simulink model "Battery_Connected_3_Phase_GridTied_Inverter_r2019a"  (R2019a)
settings: Solver=ode3  StartTime=0.0  StopTime=4  FixedStep=dtsim  RelTol=1e-3
values from neighbouring files (symbols this model uses):
  a1_lpf = 1.3601/wc_lpf    (= 4.32933276199e-05)    [Battery_Connected_3_Phase_GridTied_Inverter_Parameters.m]    (also in NonDispDGParameters.m)
  a2_lpf = 0.6165/wc_lpf2    (= 6.24645097155e-10)    [Battery_Connected_3_Phase_GridTied_Inverter_Parameters.m]    (also in NonDispDGParameters.m)
  bf = 2 * eta * wc    [Battery_Connected_3_Phase_GridTied_Inverter_Parameters.m]    (also in NonDispDGParameters.m)
  C_HV = 100e-6    (= 0.0001)    [Battery_Connected_3_Phase_GridTied_Inverter_Parameters.m]    (also in NonDispDGParameters.m; power_converters_DAB_1ph_Parameters.m)
  C_LV = 2000e-6    (= 0.002)    [Battery_Connected_3_Phase_GridTied_Inverter_Parameters.m]    (also in NonDispDGParameters.m; power_converters_DAB_1ph_Parameters.m)
  Cdc = 2 * E_Cdc / Vdc / Vdc    (= 0.00125)    [Battery_Connected_3_Phase_GridTied_Inverter_Parameters.m]    (also in NonDispDGParameters.m)
  Cf = x*Cb    (= 7.95774715459e-06)    [Battery_Connected_3_Phase_GridTied_Inverter_Parameters.m]    (also in NonDispDGParameters.m = 8.72536076817e-06)
  cf = wc * wc    (= 15791.3670417)    [Battery_Connected_3_Phase_GridTied_Inverter_Parameters.m]    (also in NonDispDGParameters.m)
  Cs_FET = inf    [Battery_Connected_3_Phase_GridTied_Inverter_Parameters.m]    (also in NonDispDGParameters.m; power_converters_DAB_1ph_Parameters.m)
  dP1 = 0.3    [Battery_Connected_3_Phase_GridTied_Inverter_Parameters.m]    (also in NonDispDGParameters.m)
  dP2 = 0.5    [Battery_Connected_3_Phase_GridTied_Inverter_Parameters.m]    (also in NonDispDGParameters.m)
  dP3 = 0.8    [Battery_Connected_3_Phase_GridTied_Inverter_Parameters.m]    (also in NonDispDGParameters.m = 0.2)
  dP4 = -0.6    [Battery_Connected_3_Phase_GridTied_Inverter_Parameters.m]    (also in NonDispDGParameters.m)
  dtsim = 5.0e-6    (= 5e-06)    [Battery_Connected_3_Phase_GridTied_Inverter_Parameters.m]    (also in NonDispDGParameters.m)
  f0 = 50    [Battery_Connected_3_Phase_GridTied_Inverter_Parameters.m]    (also in NonDispDGParameters.m)
  Fsw = 10e3    (= 10000)    [Battery_Connected_3_Phase_GridTied_Inverter_Parameters.m]    (also in NonDispDGParameters.m; power_converters_DAB_1ph_Parameters.m = 5000)
  Ia_limit = 1    [Battery_Connected_3_Phase_GridTied_Inverter_Parameters.m]    (also in NonDispDGParameters.m)
  Ib_peak = Ib*sqrt(2)    [Battery_Connected_3_Phase_GridTied_Inverter_Parameters.m]    (also in NonDispDGParameters.m)
  Ir_limit = 1    [Battery_Connected_3_Phase_GridTied_Inverter_Parameters.m]    (also in NonDispDGParameters.m)
  Ki = Kp/Ti    [Battery_Connected_3_Phase_GridTied_Inverter_Parameters.m]    (also in NonDispDGParameters.m)
  Kii = (BW_conv/w0) * Rseries_pu * w0    [Battery_Connected_3_Phase_GridTied_Inverter_Parameters.m]    (also in NonDispDGParameters.m)
  Kip = BW_P    [Battery_Connected_3_Phase_GridTied_Inverter_Parameters.m]    (also in NonDispDGParameters.m)
  Kiq = BW_Q    [Battery_Connected_3_Phase_GridTied_Inverter_Parameters.m]    (also in NonDispDGParameters.m)
  Kp = 2/A0 * KP    [Battery_Connected_3_Phase_GridTied_Inverter_Parameters.m]    (also in NonDispDGParameters.m)
  Kpi = (BW_conv/w0) * Lseries_pu    [Battery_Connected_3_Phase_GridTied_Inverter_Parameters.m]    (also in NonDispDGParameters.m)
  Kpp = BW_P * Tconv    [Battery_Connected_3_Phase_GridTied_Inverter_Parameters.m]    (also in NonDispDGParameters.m)
  Kpq = BW_Q * Tconv    [Battery_Connected_3_Phase_GridTied_Inverter_Parameters.m]    (also in NonDispDGParameters.m)
  L_Inductor = 1000e-6    (= 0.001)    [Battery_Connected_3_Phase_GridTied_Inverter_Parameters.m]    (also in NonDispDGParameters.m; power_converters_DAB_1ph_Parameters.m = 8e-06)
  Lgrid = Xgrid/w0    (= 0.00795774715459)    [Battery_Connected_3_Phase_GridTied_Inverter_Parameters.m]    (also in NonDispDGParameters.m)
  Li = Vdc/(16*fsw*delta_Ilmax)    [Battery_Connected_3_Phase_GridTied_Inverter_Parameters.m]    (also in NonDispDGParameters.m)
  Li_pu = Li/Lb    [Battery_Connected_3_Phase_GridTied_Inverter_Parameters.m]    (also in NonDispDGParameters.m)
  Lm_Tr = 100e-3    (= 0.1)    [Battery_Connected_3_Phase_GridTied_Inverter_Parameters.m]    (also in NonDispDGParameters.m; power_converters_DAB_1ph_Parameters.m = 0.00072)
  Lprim_Tr = 1e-7    (= 1e-07)    [Battery_Connected_3_Phase_GridTied_Inverter_Parameters.m]    (also in NonDispDGParameters.m; power_converters_DAB_1ph_Parameters.m = 0)
  Lsec_Tr = 1e-7    (= 1e-07)    [Battery_Connected_3_Phase_GridTied_Inverter_Parameters.m]    (also in NonDispDGParameters.m; power_converters_DAB_1ph_Parameters.m = 1.7e-05)
  ma = E_ltl*sqrt(2)/Vdc    [Battery_Connected_3_Phase_GridTied_Inverter_Parameters.m]    (also in NonDispDGParameters.m)
  Ntran = Vmv/Vlv    (= 1.9)    [Battery_Connected_3_Phase_GridTied_Inverter_Parameters.m]    (also in NonDispDGParameters.m = 1.98952879581)
  phia = 0    [Battery_Connected_3_Phase_GridTied_Inverter_Parameters.m]    (also in NonDispDGParameters.m)
  Pinit = 0    [Battery_Connected_3_Phase_GridTied_Inverter_Parameters.m]    (also in NonDispDGParameters.m)
  Pnom = 1000    [Battery_Connected_3_Phase_GridTied_Inverter_Parameters.m]    (also in NonDispDGParameters.m; power_converters_DAB_1ph_Parameters.m = 10000)
  R_DCsrc1 = 1e-7    (= 1e-07)    [Battery_Connected_3_Phase_GridTied_Inverter_Parameters.m]    (also in NonDispDGParameters.m; power_converters_DAB_1ph_Parameters.m)
  R_Inductor = 16e-3    (= 0.016)    [Battery_Connected_3_Phase_GridTied_Inverter_Parameters.m]    (also in NonDispDGParameters.m; power_converters_DAB_1ph_Parameters.m)
  RC_HV = 1e-3    (= 0.001)    [Battery_Connected_3_Phase_GridTied_Inverter_Parameters.m]    (also in NonDispDGParameters.m; power_converters_DAB_1ph_Parameters.m)
  RC_LV = 1e-3    (= 0.001)    [Battery_Connected_3_Phase_GridTied_Inverter_Parameters.m]    (also in NonDispDGParameters.m; power_converters_DAB_1ph_Parameters.m)
  Rd = 1/(3*wres*Cf)    [Battery_Connected_3_Phase_GridTied_Inverter_Parameters.m]    (also in NonDispDGParameters.m)
  Rgrid = 0.7    [Battery_Connected_3_Phase_GridTied_Inverter_Parameters.m]    (also in NonDispDGParameters.m)
  Ri = Ri_pu*Zb    [Battery_Connected_3_Phase_GridTied_Inverter_Parameters.m]    (also in NonDispDGParameters.m)
  Rm_Tr = 1e6    (= 1000000)    [Battery_Connected_3_Phase_GridTied_Inverter_Parameters.m]    (also in NonDispDGParameters.m; power_converters_DAB_1ph_Parameters.m = 10000)
  Ron_Diode = 10e-3    (= 0.01)    [Battery_Connected_3_Phase_GridTied_Inverter_Parameters.m]    (also in NonDispDGParameters.m; power_converters_DAB_1ph_Parameters.m)
  Ron_FET = 20e-3    (= 0.02)    [Battery_Connected_3_Phase_GridTied_Inverter_Parameters.m]    (also in NonDispDGParameters.m; power_converters_DAB_1ph_Parameters.m = 0.016)
  Rprim_Tr = 10e-3    (= 0.01)    [Battery_Connected_3_Phase_GridTied_Inverter_Parameters.m]    (also in NonDispDGParameters.m; power_converters_DAB_1ph_Parameters.m = 1e-06)
  Rs_FET = 1e6    (= 1000000)    [Battery_Connected_3_Phase_GridTied_Inverter_Parameters.m]    (also in NonDispDGParameters.m; power_converters_DAB_1ph_Parameters.m)
  Rsec_Tr = 10e-3    (= 0.01)    [Battery_Connected_3_Phase_GridTied_Inverter_Parameters.m]    (also in NonDispDGParameters.m; power_converters_DAB_1ph_Parameters.m = 0.043)
  Rtran_pu = 0.003    [Battery_Connected_3_Phase_GridTied_Inverter_Parameters.m]    (also in NonDispDGParameters.m)
  Sb = Pinv    (= 1000)    [Battery_Connected_3_Phase_GridTied_Inverter_Parameters.m]    (also in NonDispDGParameters.m)
  Stran = 1000    [Battery_Connected_3_Phase_GridTied_Inverter_Parameters.m]    (also in NonDispDGParameters.m)
  tinit = 0.25    [Battery_Connected_3_Phase_GridTied_Inverter_Parameters.m]    (also in NonDispDGParameters.m)
  tP1 = 0.5    [Battery_Connected_3_Phase_GridTied_Inverter_Parameters.m]    (also in NonDispDGParameters.m)
  tP2 = 1.5    [Battery_Connected_3_Phase_GridTied_Inverter_Parameters.m]    (also in NonDispDGParameters.m)
  tP3 = 2.5    [Battery_Connected_3_Phase_GridTied_Inverter_Parameters.m]    (also in NonDispDGParameters.m)
  tP4 = 3.5    [Battery_Connected_3_Phase_GridTied_Inverter_Parameters.m]    (also in NonDispDGParameters.m)
  Ts = 1e-7    (= 1e-07)    [Battery_Connected_3_Phase_GridTied_Inverter_Parameters.m]    (also in NonDispDGParameters.m; power_converters_DAB_1ph_Parameters.m)
  Turn_ratio = 15    [Battery_Connected_3_Phase_GridTied_Inverter_Parameters.m]    (also in NonDispDGParameters.m; power_converters_DAB_1ph_Parameters.m)
  Vb_peak = Vb*sqrt(2/3)    [Battery_Connected_3_Phase_GridTied_Inverter_Parameters.m]    (also in NonDispDGParameters.m)
  Vbat = 25    [Battery_Connected_3_Phase_GridTied_Inverter_Parameters.m]    (also in NonDispDGParameters.m = 24; power_converters_DAB_1ph_Parameters.m = 24)
  Vc_prime = 0.25    [Battery_Connected_3_Phase_GridTied_Inverter_Parameters.m]    (also in NonDispDGParameters.m)
  Vdc = 400    [Battery_Connected_3_Phase_GridTied_Inverter_Parameters.m]    (also in NonDispDGParameters.m)
  Vf_Diode = 4.2    [Battery_Connected_3_Phase_GridTied_Inverter_Parameters.m]    (also in NonDispDGParameters.m; power_converters_DAB_1ph_Parameters.m)
  Vlv = 200    [Battery_Connected_3_Phase_GridTied_Inverter_Parameters.m]    (also in NonDispDGParameters.m = 191)
  Vmv = 380    [Battery_Connected_3_Phase_GridTied_Inverter_Parameters.m]    (also in NonDispDGParameters.m)
  w0 = 2*pi*f0    (= 314.159265359)    [Battery_Connected_3_Phase_GridTied_Inverter_Parameters.m]    (also in NonDispDGParameters.m)
  Xtran_pu = 0.6    [Battery_Connected_3_Phase_GridTied_Inverter_Parameters.m]    (also in NonDispDGParameters.m)
undefined symbols (not defined in the file or in its folder): D11, Delta, Ion, Lg, Lithium
libraries: powerlib x48, simulink x8, powerlib_meascontrol x4, simulink_extras x2, electricdrivelib x1
(part 2 of 2)

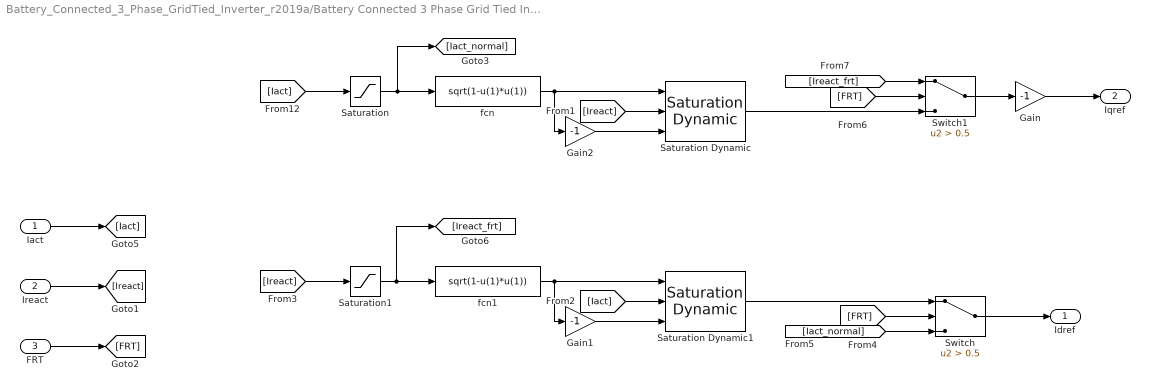
== system Battery_Connected_3_Phase_GridTied_Inverter_r2019a/Battery Connected 3 Phase Grid Tied Inverter/dq_limiter ==
  Iact : Inport
  Ireact : Inport  Port=2
  FRT : Inport  Port=3
  Gain : Gain  Gain=-1
  Gain1 : Gain  Gain=-1
  Gain2 : Gain  Gain=-1
  Saturation : Saturate  UpperLimit=1  LowerLimit=-1
  Saturation Dynamic : simulink/Discontinuities/Saturation Dynamic  OutMin=[]  OutMax=[]  OutDataTypeStr=Inherit: Same as second input  OutDataType=fixdt(1, 16)  OutScaling=2^-10  DoSatur=off
  Saturation Dynamic1 : simulink/Discontinuities/Saturation Dynamic  OutMin=[]  OutMax=[]  OutDataTypeStr=Inherit: Same as second input  OutDataType=fixdt(1, 16)  OutScaling=2^-10  DoSatur=off
  Saturation1 : Saturate  UpperLimit=1  LowerLimit=-1
  Switch : Switch  Criteria=u2 > Threshold  Threshold=0.5
  Switch1 : Switch  Criteria=u2 > Threshold  Threshold=0.5
  fcn : Fcn  Expr=sqrt(1-u(1)*u(1))
  fcn1 : Fcn  Expr=sqrt(1-u(1)*u(1))
  Idref : Outport  VectorParamsAs1DForOutWhenUnconnected=off
  Iqref : Outport  Port=2  VectorParamsAs1DForOutWhenUnconnected=off
  wires:
  fcn/1 -> Gain2/1, Saturation Dynamic/1
  Gain2/1 -> Saturation Dynamic/3
  Saturation/1 -> [Iact_normal], fcn/1
  Iact/1 -> [Iact]
  Ireact/1 -> [Ireact]
  [Iact] -> Saturation/1
  [Ireact] -> Saturation Dynamic/2
  [Iact] -> Saturation Dynamic1/2
  Gain1/1 -> Saturation Dynamic1/3
  fcn1/1 -> Gain1/1, Saturation Dynamic1/1
  [Ireact] -> Saturation1/1
  FRT/1 -> [FRT]
  [FRT] -> Switch/2
  Saturation Dynamic/1 -> Switch1/3
  Saturation1/1 -> [Ireact_frt], fcn1/1
  [Iact_normal] -> Switch/3
  Saturation Dynamic1/1 -> Switch/1
  Switch/1 -> Idref/1
  [FRT] -> Switch1/2
  [Ireact_frt] -> Switch1/1
  Switch1/1 -> Gain/1
  Gain/1 -> Iqref/1

== system Battery_Connected_3_Phase_GridTied_Inverter_r2019a/Battery Connected 3 Phase Grid Tied Inverter/dq_to_abc ==
  dq : Inport
  theta : Inport  Port=2
  Vdc : Inport  Port=3
  Divide : Product  Inputs=*/
  Mux2 : Mux  Inputs=2
  Mux3 : Mux  Inputs=3
  a : Fcn  Expr=sin(u(3))*u(1) + cos(u(3))*u(2)
  b : Fcn  Expr=sin(u(3)-2*pi/3)*u(1) + cos(u(3)-2*pi/3)*u(2)
  c : Fcn  Expr=sin(u(3)+2*pi/3)*u(1) + cos(u(3)+2*pi/3)*u(2)
  abc : Outport  VectorParamsAs1DForOutWhenUnconnected=off
  wires:
  theta/1 -> Mux2/2
  a/1 -> Mux3/1
  Mux2/1 -> b/1, c/1, a/1
  Mux3/1 -> abc/1
  c/1 -> Mux3/3
  b/1 -> Mux3/2
  Divide/1 -> Mux2/1
  dq/1 -> Divide/1
  Vdc/1 -> Divide/2

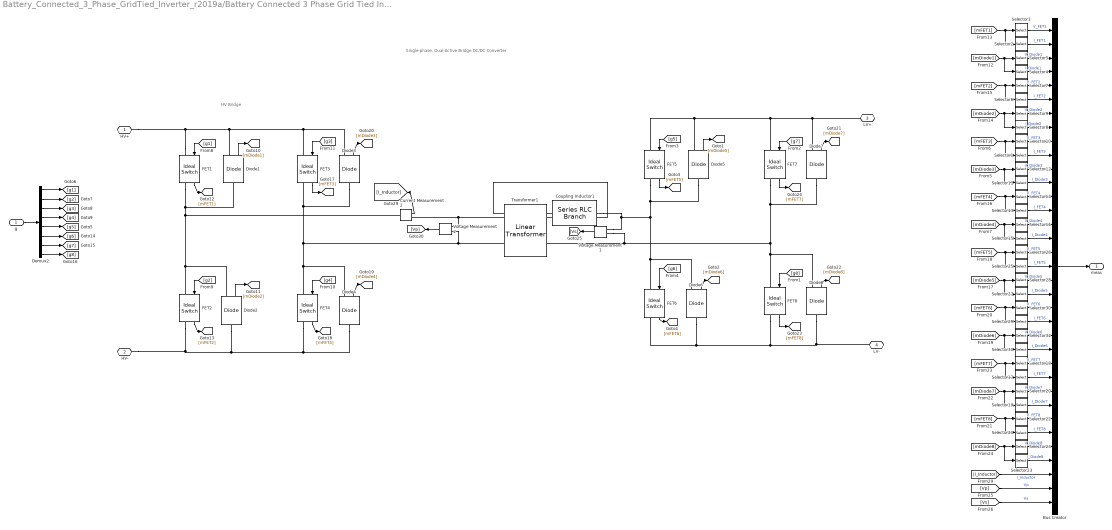
== system Battery_Connected_3_Phase_GridTied_Inverter_r2019a/Battery Connected 3 Phase Grid Tied Inverter/Dual Active Bridge/DAB2 ==
  note: HV Bridge
  note: Single-phase, Dual-Active Bridge
      | DC/DC Converter
  g : Inport  PortDimensions=8
  Bus Creator : BusCreator  Inputs=35
  Coupling Inductor1 : powerlib/Elements/Series RLC Branch  LConnTagsString=__new0  RConnTagsString=__new0  BranchType=RL  Resistance=R_Inductor  Inductance=L_Inductor  SetiL0=off  InitialCurrent=0  Capacitance=1e-6  Setx0=off  InitialVoltage=0  Measurements=None
  Current Measurement2 : powerlib/Measurements/Current Measurement  PhasorSimulation=off  OutputType=Complex  PSBequivalent=0
  Demux2 : Demux  Outputs=8
  Diode{1..8} (8 alike) : powerlib/Power Electronics/Diode  Ron=Ron_Diode  Lon=0  Vf=Vf_Diode  IC=0  UseSnubber=0  Rs=inf  Cs=inf  Measurements=on
  FET{1..8} (8 alike) : powerlib/Power Electronics/Ideal Switch  Ron=Ron_FET  Lon=0  IC=0  Rs=Rs_FET  Cs=Cs_FET  Measurements=on
  Selector{1..2,4,6,8,11,13,15,17,19,21,23,25,27,29,31} (16 alike) : Selector  InputPortWidth=2  IndexOptions=Index vector (dialog)  Indices=1  OutputSizes=1
  Selector{3,5,7,9..10,12,14,16,18,20,22,24,26,28,30,32} (16 alike) : Selector  InputPortWidth=2  IndexOptions=Index vector (dialog)  Indices=2  OutputSizes=1
  Transformer1 : powerlib/Elements/Linear Transformer  UNITS=SI  NominalPower="[ Param1_Tr(1),  Param1_Tr(2)]"  winding1="[ Param2_Tr(1),  Param2_Tr(2), Param2_Tr(3)]"  winding2="[ Param3_Tr(1),  Param3_Tr(2), Param3_Tr(3)]"  ThreeWindings=off  winding3=[3.15e+05 0.7938 0.084225]  RmLm="[ Param4_Tr(1),  Param4_Tr(2)]"  Measurements=None  DataType=on
  Voltage Measurement1 : powerlib/Measurements/Voltage Measurement  PhasorSimulation=off  OutputType=Complex  PSBequivalent=0
  Voltage Measurement2 : powerlib/Measurements/Voltage Measurement  PhasorSimulation=off  OutputType=Complex  PSBequivalent=0
  HV+ : PMIOPort  Side=Left
  HV- : PMIOPort  Port=2  Side=Left
  LV+ : PMIOPort  Port=3  Side=Right
  LV- : PMIOPort  Port=4  Side=Right
  meas : Outport  PortDimensions=35
  wires:
  Voltage Measurement2/1 -> [Vp]
  Demux2/8 -> [g8]
  Selector20/1 -> Bus Creator/27  "V_Diode7"
  Selector21/1 -> Bus Creator/30  "I_FET8"
  Selector22/1 -> Bus Creator/29  "V_FET8"
  Selector24/1 -> Bus Creator/31  "V_Diode8"
  [mDiode5] -> Selector27/1, Selector28/1
  Selector27/1 -> Bus Creator/20  "I_Diode5"
  [mFET6] -> Selector30/1, Selector29/1
  Selector23/1 -> Bus Creator/32  "I_Diode8"
  Selector32/1 -> Bus Creator/23  "V_Diode6"
  Selector26/1 -> Bus Creator/17  "V_FET5"
  Selector28/1 -> Bus Creator/19  "V_Diode5"
  Selector25/1 -> Bus Creator/18  "I_FET5"
  [mFET5] -> Selector25/1, Selector26/1
  FET3/1 -> [mFET3]
  Diode4/1 -> [mDiode4]
  FET4/1 -> [mFET4]
  Selector19/1 -> Bus Creator/28  "I_Diode7"
  FET7/1 -> [mFET7]
  Selector5/1 -> Bus Creator/3  "V_Diode1"
  [mDiode2] -> Selector8/1, Selector9/1
  [g4] -> FET4/1
  Selector4/1 -> Bus Creator/4  "I_Diode1"
  [mFET4] -> Selector14/1, Selector13/1
  Diode2/1 -> [mDiode2]
  Demux2/1 -> [g1]
  FET1/1 -> [mFET1]
  Selector18/1 -> Bus Creator/25  "V_FET7"
  Selector3/1 -> Bus Creator/1  "V_FET1"
  [mFET8] -> Selector21/1, Selector22/1
  FET2/1 -> [mFET2]
  [mDiode4] -> Selector16/1, Selector15/1
  [g1] -> FET1/1
  [g3] -> FET3/1
  Demux2/4 -> [g4]
  [mFET1] -> Selector3/1, Selector2/1
  Diode1/1 -> [mDiode1]
  Demux2/2 -> [g2]
  Diode6/1 -> [mDiode6]
  Demux2/3 -> [g3]
  Diode5/1 -> [mDiode5]
  [mDiode1] -> Selector5/1, Selector4/1
  Diode3/1 -> [mDiode3]
  Demux2/7 -> [g7]
  Selector6/1 -> Bus Creator/6  "I_FET2"
  Selector2/1 -> Bus Creator/2  "I_FET1"
  [mDiode3] -> Selector11/1, Selector12/1
  Selector13/1 -> Bus Creator/14  "I_FET4"
  Selector10/1 -> Bus Creator/9  "V_FET3"
  [mFET3] -> Selector1/1, Selector10/1
  Selector15/1 -> Bus Creator/16  "I_Diode4"
  Selector16/1 -> Bus Creator/15  "V_Diode4"
  Selector14/1 -> Bus Creator/13  "V_FET4"
  Selector30/1 -> Bus Creator/21  "V_FET6"
  [g7] -> FET7/1
  Demux2/6 -> [g6]
  [g8] -> FET8/1
  Selector9/1 -> Bus Creator/7  "V_Diode2"
  [g2] -> FET2/1
  FET6/1 -> [mFET6]
  Diode7/1 -> [mDiode7]
  [mDiode7] -> Selector20/1, Selector19/1
  Selector11/1 -> Bus Creator/12  "I_Diode3"
  Selector29/1 -> Bus Creator/22  "I_FET6"
  [mFET2] -> Selector6/1, Selector7/1
  [mDiode8] -> Selector23/1, Selector24/1
  Diode8/1 -> [mDiode8]
  FET5/1 -> [mFET5]
  Selector17/1 -> Bus Creator/26  "I_FET7"
  Selector12/1 -> Bus Creator/11  "V_Diode3"
  Current Measurement2/1 -> [I_Inductor]
  Selector1/1 -> Bus Creator/10  "I_FET3"
  Demux2/5 -> [g5]
  Selector31/1 -> Bus Creator/24  "I_Diode6"
  [mFET7] -> Selector18/1, Selector17/1
  Selector8/1 -> Bus Creator/8  "I_Diode2"
  [g5] -> FET5/1
  Selector7/1 -> Bus Creator/5  "V_FET2"
  FET8/1 -> [mFET8]
  [mDiode6] -> Selector32/1, Selector31/1
  [g6] -> FET6/1
  g/1 -> Demux2/1
  Bus Creator/1 -> meas/1
  Voltage Measurement1/1 -> [Vs]
  [I_Inductor] -> Bus Creator/33  "I_Inductor"
  [Vp] -> Bus Creator/34  "Vp"
  [Vs] -> Bus Creator/35  "Vs"
  connections:
  FET7/LConn1 -- LV+/RConn1 -- Diode7/RConn1 -- Diode5/RConn1 -- FET5/LConn1
  FET1/LConn1 -- HV+/RConn1 -- Diode3/RConn1 -- FET3/LConn1 -- Diode1/RConn1
  FET2/RConn1 -- HV-/RConn1 -- FET4/RConn1 -- Diode4/LConn1 -- Diode2/LConn1
  Diode2/RConn1 -- Current Measurement2/LConn1 -- Diode1/LConn1 -- FET1/RConn1 -- FET2/LConn1
  Diode4/RConn1 -- FET4/LConn1 -- Transformer1/LConn2 -- Voltage Measurement2/LConn2 -- FET3/RConn1 -- Diode3/LConn1
  FET6/RConn1 -- Diode6/LConn1 -- LV-/RConn1 -- Diode8/LConn1 -- FET8/RConn1
  FET7/RConn1 -- Transformer1/RConn2 -- Voltage Measurement1/LConn2 -- FET8/LConn1 -- Diode8/RConn1 -- Diode7/LConn1
  FET6/LConn1 -- Coupling Inductor1/RConn1 -- Voltage Measurement1/LConn1 -- Diode5/LConn1 -- FET5/RConn1 -- Diode6/RConn1
  Voltage Measurement2/LConn1 -- Transformer1/LConn1 -- Current Measurement2/RConn1
  Coupling Inductor1/LConn1 -- Transformer1/RConn1

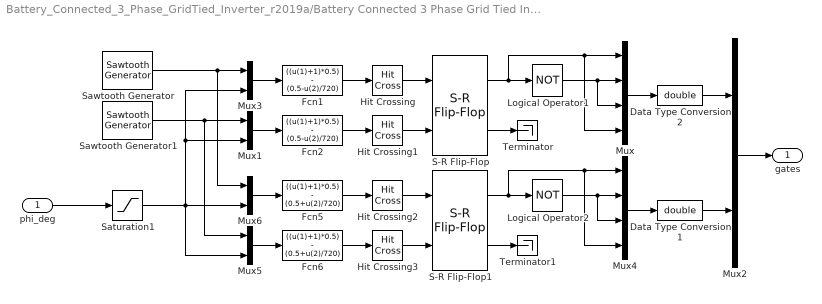
== system Battery_Connected_3_Phase_GridTied_Inverter_r2019a/Battery Connected 3 Phase Grid Tied Inverter/Dual Active Bridge/Pulses_Generator ==
  phi_deg : Inport
  Data Type Conversion1 : DataTypeConversion  OutDataTypeStr=double
  Data Type Conversion2 : DataTypeConversion  OutDataTypeStr=double
  Fcn1 : Fcn  Expr=((u(1)+1)*0.5) - (0.5-u(2)/720)
  Fcn2 : Fcn  Expr=((u(1)+1)*0.5) - (0.5-u(2)/720)
  Fcn5 : Fcn  Expr=((u(1)+1)*0.5) - (0.5+u(2)/720)
  Fcn6 : Fcn  Expr=((u(1)+1)*0.5) - (0.5+u(2)/720)
  Hit Crossing{,1..3} (4 alike) : HitCross  HitCrossingDirection=rising
  Logical Operator1 : Logic  Operator=NOT  AllPortsSameDT=off  OutDataTypeStr=boolean
  Logical Operator2 : Logic  Operator=NOT  AllPortsSameDT=off  OutDataTypeStr=boolean
  Mux : Mux
  Mux{1,3,5..6} (4 alike) : Mux  Inputs=2
  Mux2 : Mux  Inputs=[4,4]
  Mux4 : Mux
  S-R Flip-Flop : simulink_extras/Flip Flops/S-R Flip-Flop  initial_condition=0
  S-R Flip-Flop1 : simulink_extras/Flip Flops/S-R Flip-Flop  initial_condition=0
  Saturation1 : Saturate  UpperLimit=180  LowerLimit=-180
  Sawtooth Generator : powerlib_meascontrol/Pulse & Signal Generators/Sawtooth Generator  Freq=Fsw  Phase=0  Ts=0
  Sawtooth Generator1 : powerlib_meascontrol/Pulse & Signal Generators/Sawtooth Generator  Freq=Fsw  Phase=180  Ts=0
  Terminator : Terminator
  Terminator1 : Terminator
  gates : Outport
  wires:
  Mux2/1 -> gates/1
  Logical Operator1/1 -> Mux/2, Mux/3
  phi_deg/1 -> Saturation1/1
  Sawtooth Generator/1 -> Mux6/1, Mux3/1
  Fcn1/1 -> Hit Crossing/1
  Fcn2/1 -> Hit Crossing1/1
  Hit Crossing/1 -> S-R Flip-Flop/1
  Hit Crossing1/1 -> S-R Flip-Flop/2
  S-R Flip-Flop/1 -> Mux/4, Mux/1, Logical Operator1/1
  S-R Flip-Flop/2 -> Terminator/1
  Mux/1 -> Data Type Conversion2/1
  Data Type Conversion2/1 -> Mux2/1
  Data Type Conversion1/1 -> Mux2/2
  Mux3/1 -> Fcn1/1
  Mux1/1 -> Fcn2/1
  Sawtooth Generator1/1 -> Mux5/1, Mux1/1
  Saturation1/1 -> Mux6/2, Mux5/2, Mux1/2, Mux3/2
  Mux5/1 -> Fcn6/1
  Mux6/1 -> Fcn5/1
  Mux4/1 -> Data Type Conversion1/1
  S-R Flip-Flop1/2 -> Terminator1/1
  S-R Flip-Flop1/1 -> Logical Operator2/1, Mux4/1, Mux4/4
  Hit Crossing3/1 -> S-R Flip-Flop1/2
  Hit Crossing2/1 -> S-R Flip-Flop1/1
  Fcn6/1 -> Hit Crossing3/1
  Fcn5/1 -> Hit Crossing2/1
  Logical Operator2/1 -> Mux4/3, Mux4/2

== system Battery_Connected_3_Phase_GridTied_Inverter_r2019a/Battery Connected 3 Phase Grid Tied Inverter/LPF/LPF_abc ==
  X : Inport
  Demux : Demux  Outputs=3
  Mux : Mux  Inputs=3
  measurement_LPF : TransferFcn  Denominator=[a2_lpf a1_lpf 1]
  measurement_LPF1 : TransferFcn  Denominator=[a2_lpf a1_lpf 1]
  measurement_LPF2 : TransferFcn  Denominator=[a2_lpf a1_lpf 1]
  X_f : Outport  VectorParamsAs1DForOutWhenUnconnected=off
  wires:
  X/1 -> Demux/1
  measurement_LPF/1 -> Mux/1
  Demux/1 -> measurement_LPF/1
  Mux/1 -> X_f/1
  measurement_LPF2/1 -> Mux/3
  Demux/3 -> measurement_LPF2/1
  measurement_LPF1/1 -> Mux/2
  Demux/2 -> measurement_LPF1/1

== system Battery_Connected_3_Phase_GridTied_Inverter_r2019a/Battery Connected 3 Phase Grid Tied Inverter/LPF/LPF_abc1 ==
  X : Inport
  Demux : Demux  Outputs=3
  Mux : Mux  Inputs=3
  measurement_LPF : TransferFcn  Denominator=[a2_lpf a1_lpf 1]
  measurement_LPF1 : TransferFcn  Denominator=[a2_lpf a1_lpf 1]
  measurement_LPF2 : TransferFcn  Denominator=[a2_lpf a1_lpf 1]
  X_f : Outport  VectorParamsAs1DForOutWhenUnconnected=off
  wires:
  X/1 -> Demux/1
  measurement_LPF/1 -> Mux/1
  Demux/1 -> measurement_LPF/1
  Mux/1 -> X_f/1
  measurement_LPF2/1 -> Mux/3
  Demux/3 -> measurement_LPF2/1
  measurement_LPF1/1 -> Mux/2
  Demux/2 -> measurement_LPF1/1

== system Battery_Connected_3_Phase_GridTied_Inverter_r2019a/Battery Connected 3 Phase Grid Tied Inverter/LPF/LPF_abc2 ==
  X : Inport
  Demux : Demux  Outputs=3
  Mux : Mux  Inputs=3
  measurement_LPF : TransferFcn  Denominator=[a2_lpf a1_lpf 1]
  measurement_LPF1 : TransferFcn  Denominator=[a2_lpf a1_lpf 1]
  measurement_LPF2 : TransferFcn  Denominator=[a2_lpf a1_lpf 1]
  X_f : Outport  VectorParamsAs1DForOutWhenUnconnected=off
  wires:
  X/1 -> Demux/1
  measurement_LPF/1 -> Mux/1
  Demux/1 -> measurement_LPF/1
  Mux/1 -> X_f/1
  measurement_LPF2/1 -> Mux/3
  Demux/3 -> measurement_LPF2/1
  measurement_LPF1/1 -> Mux/2
  Demux/2 -> measurement_LPF1/1

== system Battery_Connected_3_Phase_GridTied_Inverter_r2019a/Battery Connected 3 Phase Grid Tied Inverter/LPF/LPF_abc3 ==
  X : Inport
  Demux : Demux  Outputs=3
  Mux : Mux  Inputs=3
  measurement_LPF : TransferFcn  Denominator=[a2_lpf a1_lpf 1]
  measurement_LPF1 : TransferFcn  Denominator=[a2_lpf a1_lpf 1]
  measurement_LPF2 : TransferFcn  Denominator=[a2_lpf a1_lpf 1]
  X_f : Outport  VectorParamsAs1DForOutWhenUnconnected=off
  wires:
  X/1 -> Demux/1
  measurement_LPF/1 -> Mux/1
  Demux/1 -> measurement_LPF/1
  Mux/1 -> X_f/1
  measurement_LPF2/1 -> Mux/3
  Demux/3 -> measurement_LPF2/1
  measurement_LPF1/1 -> Mux/2
  Demux/2 -> measurement_LPF1/1

== system Battery_Connected_3_Phase_GridTied_Inverter_r2019a/Battery Connected 3 Phase Grid Tied Inverter/Measurement/PLL ==
  Uabc : Inport
  Constant2 : Constant  Value=w0
  Constant3 : Constant  Value=2*pi
  Demux1 : Demux  Outputs=2
  Gain2 : Gain  Gain=Kp
  Gain3 : Gain  Gain=Ki
  Integrator2 : Integrator
  Integrator3 : Integrator
  Math Function1 : Math  Operator=rem  SaturateOnIntegerOverflow=on
  Sum3 : Sum  Inputs=|++
  Sum4 : Sum  Inputs=|++
  Terminator : Terminator
  abc_to_dq : Subsystem
  Angle : Outport  VectorParamsAs1DForOutWhenUnconnected=off
  w : Outport  Port=2  VectorParamsAs1DForOutWhenUnconnected=off
  Vdpos : Outport  Port=3  VectorParamsAs1DForOutWhenUnconnected=off
  wires:
  abc_to_dq/1(Vdqpos) -> Demux1/1
  Uabc/1 -> abc_to_dq/1(Uabc)
  Constant2/1 -> Sum3/2
  Demux1/1 -> Vdpos/1
  Integrator2/1 -> Math Function1/1
  Demux1/2 -> Gain2/1, Gain3/1
  Sum4/1 -> w/1, Integrator2/1
  Gain3/1 -> Integrator3/1
  abc_to_dq/2(Vdqneg) -> Terminator/1
  Gain2/1 -> Sum4/2
  Constant3/1 -> Math Function1/2
  Sum3/1 -> Sum4/1
  Integrator3/1 -> Sum3/1
  Math Function1/1 -> abc_to_dq/2(wt), Angle/1

== system Battery_Connected_3_Phase_GridTied_Inverter_r2019a/Battery Connected 3 Phase Grid Tied Inverter/Measurement/abc_to_dq ==
  abc : Inport
  theta : Inport  Port=2
  Gain1 : Gain  Gain=2/3
  Mux2 : Mux  Inputs=2
  Mux3 : Mux  Inputs=2
  d : Fcn  Expr=sin(u(4))*u(1) + sin(u(4)-2*pi/3)*u(2) + sin(u(4)+2*pi/3)*u(3)
  q : Fcn  Expr=cos(u(4))*u(1) + cos(u(4)-2*pi/3)*u(2) + cos(u(4)+2*pi/3)*u(3)
  dq : Outport  VectorParamsAs1DForOutWhenUnconnected=off
  wires:
  Mux3/1 -> Gain1/1
  theta/1 -> Mux2/2
  abc/1 -> Mux2/1
  Gain1/1 -> dq/1
  Mux2/1 -> d/1, q/1
  d/1 -> Mux3/1
  q/1 -> Mux3/2

== system Battery_Connected_3_Phase_GridTied_Inverter_r2019a/Battery Connected 3 Phase Grid Tied Inverter/Measurement/abc_to_dq1 ==
  abc : Inport
  theta : Inport  Port=2
  Gain1 : Gain  Gain=2/3
  Mux2 : Mux  Inputs=2
  Mux3 : Mux  Inputs=2
  d : Fcn  Expr=sin(u(4))*u(1) + sin(u(4)-2*pi/3)*u(2) + sin(u(4)+2*pi/3)*u(3)
  q : Fcn  Expr=cos(u(4))*u(1) + cos(u(4)-2*pi/3)*u(2) + cos(u(4)+2*pi/3)*u(3)
  dq : Outport  VectorParamsAs1DForOutWhenUnconnected=off
  wires:
  Mux3/1 -> Gain1/1
  theta/1 -> Mux2/2
  abc/1 -> Mux2/1
  Gain1/1 -> dq/1
  Mux2/1 -> d/1, q/1
  d/1 -> Mux3/1
  q/1 -> Mux3/2

== system Battery_Connected_3_Phase_GridTied_Inverter_r2019a/Battery Connected 3 Phase Grid Tied Inverter/Measurement/abc_to_dq2 ==
  abc : Inport
  theta : Inport  Port=2
  Gain1 : Gain  Gain=2/3
  Mux2 : Mux  Inputs=2
  Mux3 : Mux  Inputs=2
  d : Fcn  Expr=sin(u(4))*u(1) + sin(u(4)-2*pi/3)*u(2) + sin(u(4)+2*pi/3)*u(3)
  q : Fcn  Expr=cos(u(4))*u(1) + cos(u(4)-2*pi/3)*u(2) + cos(u(4)+2*pi/3)*u(3)
  dq : Outport  VectorParamsAs1DForOutWhenUnconnected=off
  wires:
  Mux3/1 -> Gain1/1
  theta/1 -> Mux2/2
  abc/1 -> Mux2/1
  Gain1/1 -> dq/1
  Mux2/1 -> d/1, q/1
  d/1 -> Mux3/1
  q/1 -> Mux3/2

== system Battery_Connected_3_Phase_GridTied_Inverter_r2019a/Battery Connected 3 Phase Grid Tied Inverter/Measurement/abc_to_dq3 ==
  abc : Inport
  theta : Inport  Port=2
  Gain1 : Gain  Gain=2/3
  Mux2 : Mux  Inputs=2
  Mux3 : Mux  Inputs=2
  d : Fcn  Expr=sin(u(4))*u(1) + sin(u(4)-2*pi/3)*u(2) + sin(u(4)+2*pi/3)*u(3)
  q : Fcn  Expr=cos(u(4))*u(1) + cos(u(4)-2*pi/3)*u(2) + cos(u(4)+2*pi/3)*u(3)
  dq : Outport  VectorParamsAs1DForOutWhenUnconnected=off
  wires:
  Mux3/1 -> Gain1/1
  theta/1 -> Mux2/2
  abc/1 -> Mux2/1
  Gain1/1 -> dq/1
  Mux2/1 -> d/1, q/1
  d/1 -> Mux3/1
  q/1 -> Mux3/2

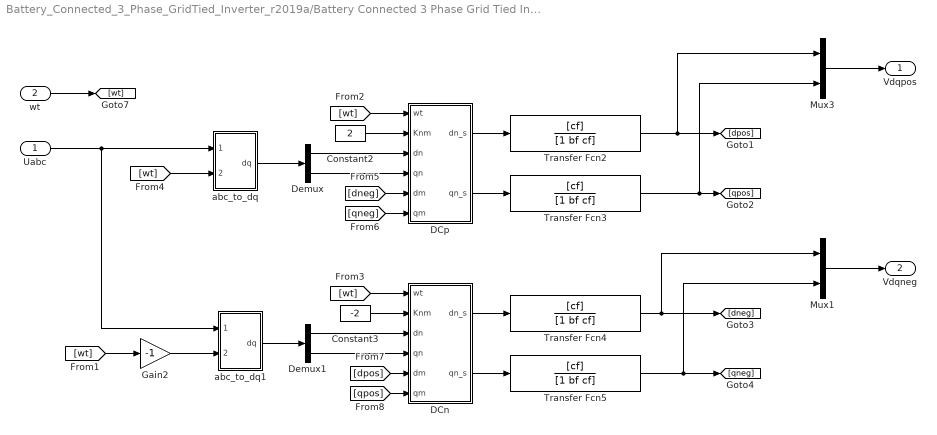
== system Battery_Connected_3_Phase_GridTied_Inverter_r2019a/Battery Connected 3 Phase Grid Tied Inverter/Measurement/PLL/abc_to_dq ==
  Uabc : Inport
  wt : Inport  Port=2
  Constant2 : Constant  Value=2
  Constant3 : Constant  Value=-2
  DCn : Subsystem
  DCp : Subsystem
  Demux : Demux  Outputs=2
  Demux1 : Demux  Outputs=2
  Gain2 : Gain  Gain=-1
  Mux1 : Mux  Inputs=2
  Mux3 : Mux  Inputs=2
  Transfer Fcn{2..5} (4 alike) : TransferFcn  Numerator=[cf]  Denominator=[1 bf cf]
  abc_to_dq : Subsystem
  abc_to_dq1 : Subsystem
  Vdqpos : Outport  VectorParamsAs1DForOutWhenUnconnected=off
  Vdqneg : Outport  Port=2  VectorParamsAs1DForOutWhenUnconnected=off
  wires:
  Demux1/1 -> DCn/3(dn)
  Transfer Fcn5/1 -> Mux1/2, [qneg]
  Gain2/1 -> abc_to_dq1/2(theta)
  Demux1/2 -> DCn/4(qn)
  Uabc/1 -> abc_to_dq1/1(abc), abc_to_dq/1(abc)
  Transfer Fcn3/1 -> Mux3/2, [qpos]
  Mux3/1 -> Vdqpos/1
  Transfer Fcn2/1 -> [dpos], Mux3/1
  [wt] -> DCp/1(wt)
  [wt] -> Gain2/1
  Transfer Fcn4/1 -> Mux1/1, [dneg]
  Demux/2 -> DCp/4(qn)
  DCn/2(qn_s) -> Transfer Fcn5/1
  wt/1 -> [wt]
  Demux/1 -> DCp/3(dn)
  [qneg] -> DCp/6(qm)
  DCp/2(qn_s) -> Transfer Fcn3/1
  [dneg] -> DCp/5(dm)
  [qpos] -> DCn/6(qm)
  Constant2/1 -> DCp/2(Knm)
  [dpos] -> DCn/5(dm)
  Mux1/1 -> Vdqneg/1
  Constant3/1 -> DCn/2(Knm)
  [wt] -> DCn/1(wt)
  DCn/1(dn_s) -> Transfer Fcn4/1
  DCp/1(dn_s) -> Transfer Fcn2/1
  [wt] -> abc_to_dq/2(theta)
  abc_to_dq/1(dq) -> Demux/1
  abc_to_dq1/1(dq) -> Demux1/1

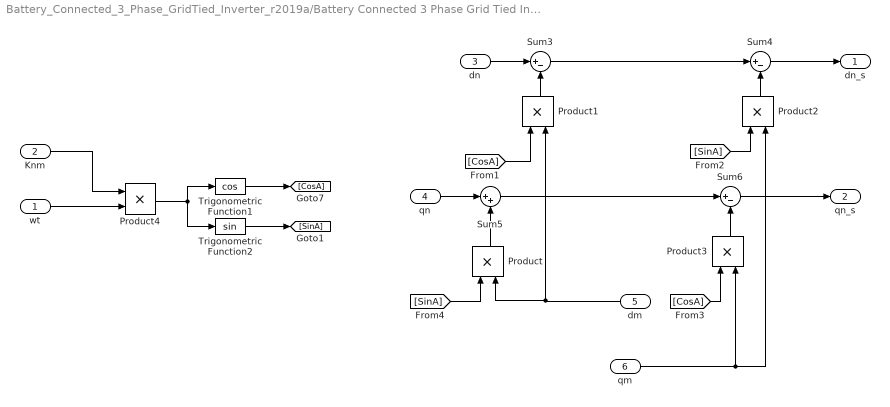
== system Battery_Connected_3_Phase_GridTied_Inverter_r2019a/Battery Connected 3 Phase Grid Tied Inverter/Measurement/PLL/abc_to_dq/DCn ==
  wt : Inport
  Knm : Inport  Port=2
  dn : Inport  Port=3
  qn : Inport  Port=4
  dm : Inport  Port=5
  qm : Inport  Port=6
  Product{,1..4} (5 alike) : Product
  Sum3 : Sum  Inputs=|+-
  Sum4 : Sum  Inputs=|+-
  Sum5 : Sum  Inputs=|++
  Sum6 : Sum  Inputs=|+-
  Trigonometric Function1 : Trigonometry  Operator=cos
  Trigonometric Function2 : Trigonometry
  dn_s : Outport  VectorParamsAs1DForOutWhenUnconnected=off
  qn_s : Outport  Port=2  VectorParamsAs1DForOutWhenUnconnected=off
  wires:
  dn/1 -> Sum3/1
  Product4/1 -> Trigonometric Function2/1, Trigonometric Function1/1
  Sum4/1 -> dn_s/1
  dm/1 -> Product1/2, Product/2
  Sum3/1 -> Sum4/1
  [SinA] -> Product2/1
  Product1/1 -> Sum3/2
  wt/1 -> Product4/2
  qm/1 -> Product2/2, Product3/2
  Product/1 -> Sum5/2
  qn/1 -> Sum5/1
  [SinA] -> Product/1
  Product2/1 -> Sum4/2
  Product3/1 -> Sum6/2
  Trigonometric Function1/1 -> [CosA]
  Trigonometric Function2/1 -> [SinA]
  Sum5/1 -> Sum6/1
  [CosA] -> Product3/1
  [CosA] -> Product1/1
  Knm/1 -> Product4/1
  Sum6/1 -> qn_s/1

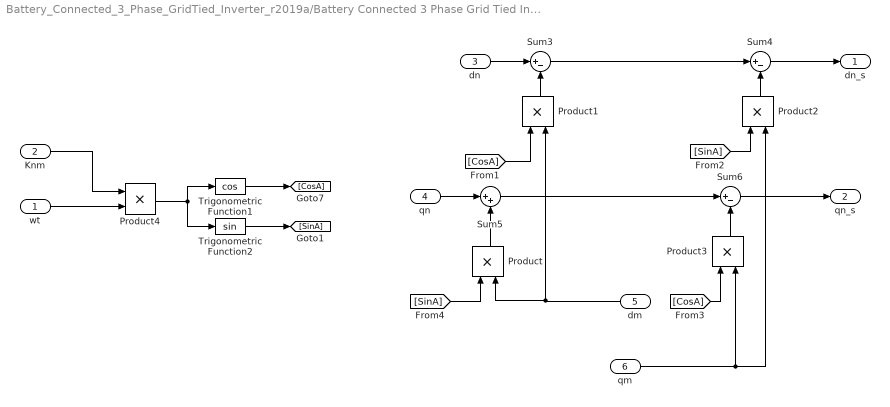
== system Battery_Connected_3_Phase_GridTied_Inverter_r2019a/Battery Connected 3 Phase Grid Tied Inverter/Measurement/PLL/abc_to_dq/DCp ==
  wt : Inport
  Knm : Inport  Port=2
  dn : Inport  Port=3
  qn : Inport  Port=4
  dm : Inport  Port=5
  qm : Inport  Port=6
  Product{,1..4} (5 alike) : Product
  Sum3 : Sum  Inputs=|+-
  Sum4 : Sum  Inputs=|+-
  Sum5 : Sum  Inputs=|++
  Sum6 : Sum  Inputs=|+-
  Trigonometric Function1 : Trigonometry  Operator=cos
  Trigonometric Function2 : Trigonometry
  dn_s : Outport  VectorParamsAs1DForOutWhenUnconnected=off
  qn_s : Outport  Port=2  VectorParamsAs1DForOutWhenUnconnected=off
  wires:
  dn/1 -> Sum3/1
  Product4/1 -> Trigonometric Function2/1, Trigonometric Function1/1
  Sum4/1 -> dn_s/1
  dm/1 -> Product1/2, Product/2
  Sum3/1 -> Sum4/1
  [SinA] -> Product2/1
  Product1/1 -> Sum3/2
  wt/1 -> Product4/2
  qm/1 -> Product2/2, Product3/2
  Product/1 -> Sum5/2
  qn/1 -> Sum5/1
  [SinA] -> Product/1
  Product2/1 -> Sum4/2
  Product3/1 -> Sum6/2
  Trigonometric Function1/1 -> [CosA]
  Trigonometric Function2/1 -> [SinA]
  Sum5/1 -> Sum6/1
  [CosA] -> Product3/1
  [CosA] -> Product1/1
  Knm/1 -> Product4/1
  Sum6/1 -> qn_s/1

== system Battery_Connected_3_Phase_GridTied_Inverter_r2019a/Battery Connected 3 Phase Grid Tied Inverter/Measurement/PLL/abc_to_dq/abc_to_dq ==
  abc : Inport
  theta : Inport  Port=2
  Gain1 : Gain  Gain=2/3
  Mux2 : Mux  Inputs=2
  Mux3 : Mux  Inputs=2
  d : Fcn  Expr=sin(u(4))*u(1) + sin(u(4)-2*pi/3)*u(2) + sin(u(4)+2*pi/3)*u(3)
  q : Fcn  Expr=cos(u(4))*u(1) + cos(u(4)-2*pi/3)*u(2) + cos(u(4)+2*pi/3)*u(3)
  dq : Outport  VectorParamsAs1DForOutWhenUnconnected=off
  wires:
  Mux3/1 -> Gain1/1
  theta/1 -> Mux2/2
  abc/1 -> Mux2/1
  Gain1/1 -> dq/1
  d/1 -> Mux3/1
  Mux2/1 -> q/1, d/1
  q/1 -> Mux3/2

== system Battery_Connected_3_Phase_GridTied_Inverter_r2019a/Battery Connected 3 Phase Grid Tied Inverter/Measurement/PLL/abc_to_dq/abc_to_dq1 ==
  abc : Inport
  theta : Inport  Port=2
  Gain1 : Gain  Gain=2/3
  Mux2 : Mux  Inputs=2
  Mux3 : Mux  Inputs=2
  d : Fcn  Expr=sin(u(4))*u(1) + sin(u(4)-2*pi/3)*u(2) + sin(u(4)+2*pi/3)*u(3)
  q : Fcn  Expr=cos(u(4))*u(1) + cos(u(4)-2*pi/3)*u(2) + cos(u(4)+2*pi/3)*u(3)
  dq : Outport  VectorParamsAs1DForOutWhenUnconnected=off
  wires:
  Mux3/1 -> Gain1/1
  theta/1 -> Mux2/2
  abc/1 -> Mux2/1
  Gain1/1 -> dq/1
  d/1 -> Mux3/1
  Mux2/1 -> q/1, d/1
  q/1 -> Mux3/2
